simulink model "LLC_fast_PI_MOS"  (R2024a)
settings: Solver=FixedStepDiscrete  StartTime=0.0  StopTime=0.3  FixedStep=Ts_Power  RelTol=1e-3  EnableMultiTasking=on
values from neighbouring files (symbols this model uses):
  Co = 560e-6    (= 0.00056)    [LLC_Data.m]    (also in LLC_Reverse_Data.m)
  Cr = 140e-9    (= 1.4e-07)    [LLC_Data.m]    (also in LLC_Reverse_Data.m)
  fs_LCC_max = 250e3    (= 250000)    [LLC_Data.m]    (also in LLC_Reverse_Data.m)
  fs_LCC_min = 40e3    (= 40000)    [LLC_Data.m]    (also in LLC_Reverse_Data.m)
  Ki_LLC = 500e3    (= 500000)    [LLC_Data.m]    (also in LLC_Reverse_Data.m)
  Kp_LLC = 5e3    (= 5000)    [LLC_Data.m]    (also in LLC_Reverse_Data.m)
  Lm = 100e-6    (= 0.0001)    [LLC_Data.m]    (also in LLC_Reverse_Data.m)
  Lr = 20e-6    (= 2e-05)    [LLC_Data.m]    (also in LLC_Reverse_Data.m)
  Np = 11    [LLC_Data.m]    (also in LLC_Reverse_Data.m)
  Ns = 10    [LLC_Data.m]    (also in LLC_Reverse_Data.m)
  Ro = Vo_nom^2/Po_nom    (= 19.6363636364)    [LLC_Data.m]    (also in LLC_Reverse_Data.m)
  Ts_Control = 10e-6    (= 1e-05)    [LLC_Data.m]    (also in LLC_Reverse_Data.m)
  Ts_Power = 50e-9    (= 5e-08)    [LLC_Data.m]    (also in LLC_Reverse_Data.m)
  V_o_max = 450    [LLC_Data.m]    (also in LLC_Reverse_Data.m)
  V_o_min = 275    [LLC_Data.m]    (also in LLC_Reverse_Data.m)
  Vdc_in = 400    [LLC_Data.m]    (also in LLC_Reverse_Data.m)
undefined symbols (not defined in the file or in its folder): DiscIntNeverNeededParam
libraries: spsMosfetLib x8, spsVoltageMeasurementLib x5, spsOnDelayLib x4, spsSeriesRLCBranchLib x3, spsCurrentMeasurementLib x3, spsDCVoltageSourceLib x1, slpidlib x1, spsLinearTransformerLib x1, spspowerguiLib x1
settings Model: SimulationMode=accelerator  Creator=LWYohann  LastModifiedBy=LWYohann

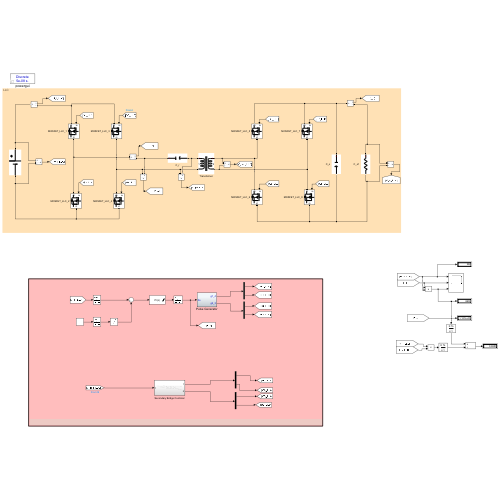
[thumbnail: Simulink's stored preview of the top-level diagram]
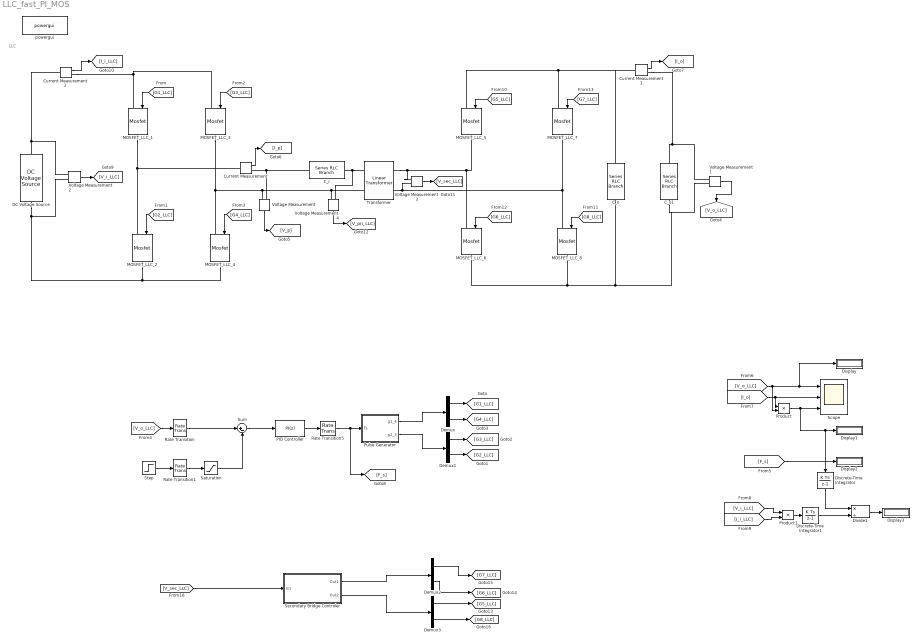
== system LLC_fast_PI_MOS ==
  note: LLC
  C_o : spsSeriesRLCBranchLib/Series RLC Branch  LConnTagsString=__new0  RConnTagsString=__new0  BranchType=C  Resistance=1  Inductance=1e-3  SetiL0=off  InitialCurrent=0  Capacitance=Co  Setx0=on  InitialVoltage=Vo_nom  Measurements=None
  C_o1 : spsSeriesRLCBranchLib/Series RLC Branch  LConnTagsString=__new0  RConnTagsString=__new0  BranchType=R  Resistance=Ro  Inductance=1e-3  SetiL0=off  InitialCurrent=0  Capacitance=Co  Setx0=on  InitialVoltage=375  Measurements=None
  C_r : spsSeriesRLCBranchLib/Series RLC Branch  LConnTagsString=__new0  RConnTagsString=__new0  BranchType=C  Resistance=1  Inductance=1e-3  SetiL0=off  InitialCurrent=0  Capacitance=Cr  Setx0=off  InitialVoltage=0  Measurements=None
  Current Measurement : spsCurrentMeasurementLib/Current Measurement  PhasorSimulation=off  OutputType=Complex  PSBequivalent=0
  Current Measurement1 : spsCurrentMeasurementLib/Current Measurement  PhasorSimulation=off  OutputType=Complex  PSBequivalent=0
  Current Measurement2 : spsCurrentMeasurementLib/Current Measurement  PhasorSimulation=off  OutputType=Complex  PSBequivalent=0
  DC Voltage Source : spsDCVoltageSourceLib/DC Voltage Source  Amplitude=Vdc_in  Measurements=None
  Demux{,1..3} (4 alike) : Demux  Outputs=2
  Discrete-Time Integrator : DiscreteIntegrator  SampleTime=Ts_Power  ICPrevOutput=DiscIntNeverNeededParam  ICPrevScaledInput=DiscIntNeverNeededParam
  Discrete-Time Integrator1 : DiscreteIntegrator  SampleTime=Ts_Power  ICPrevOutput=DiscIntNeverNeededParam  ICPrevScaledInput=DiscIntNeverNeededParam
  Display{,1..3} (4 alike) : Display
      Display3 settings: Decimation=2
  Divide1 : Product  Inputs=*/
  MOSFET_LLC_{1..8} (8 alike) : spsMosfetLib/Mosfet  Ron=Ron_FET  Lon=0  Rd=Ron_Diode  Vfd=Vf  IC=0  Rs=1e6  Cs=inf  Measurements=off
  PID Controller : slpidlib/PID Controller  Controller=PI  Form=Parallel  TimeDomain=Discrete-time  UseExternalTs=off  SampleTime=Ts_Control  IntegratorMethod=Forward Euler  FilterMethod=Forward Euler  ControllerParametersSource=internal  P=Kp_LLC  I=Ki_LLC  UseKiTs=off  D=0  UseExternalDerivativeSource=off  N=100  UseFilter=on  TunerSelectOption=Transfer Function Based (PID Tuner App)  InitialConditionSource=internal  InitialConditionForIntegrator=fr  InitialConditionForFilter=0  DifferentiatorICPrevScaledInput=0  ExternalReset=none  TrackingMode=off  Kt=1  LimitOutput=on  SatLimitsSource=internal  UpperSaturationLimit=fs_LCC_max  LowerSaturationLimit=fs_LCC_min  LinearizeAsGain=on  AntiWindupMode=none  Kb=1  LimitIntegrator=on  UpperIntegratorSaturationLimit=fs_LCC_max  LowerIntegratorSaturationLimit=fs_LCC_min  POutMin=[]  POutMax=[]  IOutMin=[]  IOutMax=[]  DOutMin=[]  DOutMax=[]  NOutMin=[]  NOutMax=[]  SumOutMin=[]  SumOutMax=[]  SaturationOutMin=[]  SaturationOutMax=[]  PParamMin=[]  PParamMax=[]  IParamMin=[]  IParamMax=[]  DParamMin=[]  DParamMax=[]  NParamMin=[]  NParamMax=[]  KbParamMin=[]  KbParamMax=[]  KtParamMin=[]  KtParamMax=[]  KbOutMin=[]  KbOutMax=[]  KtOutMin=[]  KtOutMax=[]  IntegratorOutMin=[]  IntegratorOutMax=[]  FilterOutMin=[]  FilterOutMax=[]  SumI1OutMin=[]  SumI1OutMax=[]  SumI2OutMin=[]  SumI2OutMax=[]  SumI3OutMin=[]  SumI3OutMax=[]  SumI4OutMin=[]  SumI4OutMax=[]  SumDOutMin=[]  SumDOutMax=[]  DifferentiatorOutMin=[]  DifferentiatorOutMax=[]  FilterDiffOutCoefMin=[]  FilterDiffOutCoefMax=[]  ReciprocalOutMin=[]  ReciprocalOutMax=[]  SumDenOutMin=[]  SumDenOutMax=[]  SumNumOutMin=[]  SumNumOutMax=[]  DivideOutMin=[]  DivideOutMax=[]  UdiffTsProdOutMin=[]  UdiffTsProdOutMax=[]  NTsProdOutMin=[]  NTsProdOutMax=[]  UintegralTsProdOutMin=[]  UintegralTsProdOutMax=[]  UngainTsProdOutMin=[]  UngainTsProdOutMax=[]  ClampingZeroOutDataTypeStr=Inherit: Inherit via back propagation  ClampingZeroOutMin=[]  ClampingZeroOutMax=[]  FilterDenConstantOutDataTypeStr=Inherit: Inherit via back propagation  FilterDenConstantOutMin=[]  FilterDenConstantOutMax=[]  PCopyOutDataTypeStr=Inherit: Inherit via back propagation  PCopyOutMin=[]  PCopyOutMax=[]  NCopyOutDataTypeStr=Inherit: Inherit via back propagation  NCopyOutMin=[]  NCopyOutMax=[]  IntegratorContinuousStateAttributes=''  IntegratorStateMustResolveToSignalObject=off  IntegratorRTWStateStorageClass=Auto  FilterContinuousStateAttributes=''  FilterStateMustResolveToSignalObject=off  FilterRTWStateStorageClass=Auto  ParallelPVariant=InternalParameters  IdealPVariant=Disabled  IVariant=InternalParameters  DVariant=Disabled  IntegratorVariant=Discrete  SatVariant=Enabled  AWVariant=Passthrough  PCopyVariant=Disabled  TRVariant=Disabled  FdbkBlocksVariant=Forward  IdealPFdbkVariant=Disabled  SatFdbkVariant=Disabled  DerivativeFilterVariant=Disabled  NVariant=Disabled  NCopyVariant=Disabled_SignalSpec  FilterICVariant=Disabled  IntegratorICVariant=InternalICs  ExternalResetVariant=Disabled  TRSumVariant=Passthrough  SumFdbkVariant=Disabled  SumVariant=Sum_PI  TsampFilterVariant=InternalTs  TsampNgainVariant=Passthrough  TsampIntegralVariant=Disabled_SignalSpec  ExternalSaturationOutDataTypeStr=Inherit: Same as second input  DerivativeSourceVariant=Disabled
  Product : Product
  Product1 : Product
  Pulse Generator : Subsystem
  Rate Transition : RateTransition  OutPortSampleTime=Ts_Control
  Rate Transition1 : RateTransition  OutPortSampleTime=Ts_Control
  Rate Transition5 : RateTransition  InitialCondition=fs_LCC_min  OutPortSampleTime=Ts_Power
  Saturation : Saturate  UpperLimit=V_o_max  LowerLimit=V_o_min
  Scope : Scope  NumInputPorts=3
  Secondary Bridge Controler : Subsystem
  Step : Step  Time=0.1  Before=275  After=360  SampleTime=Ts_Power
  Sum : Sum  Inputs=|+-
  Transformer : spsLinearTransformerLib/Linear Transformer  UNITS=SI  NominalPower=[ 6.6e3 100e3 ]  winding1="[Np   1e-2 Lr]"  winding2="[Ns  1e-2  1e-8 ]"  ThreeWindings=off  winding3=[3.15e+05 0.7938 0.084225]  RmLm=[1e4 Lm]  Measurements=None  DataType=on
  Voltage Measurement{,1..4} (5 alike) : spsVoltageMeasurementLib/Voltage Measurement  PhasorSimulation=off  OutputType=Complex  PSBequivalent=0
  powergui : spspowerguiLib/powergui  Priority=1  SimulationMode=Discrete  SampleTime=Ts_Power  frequency=60  Iterations=50  frequencyindice=0  Pbase=100e6  ErrMax=1e-4  UnitsV=kV  UnitsW=MW  buscounter=0  FunctionMessages=off  echomessages=off  EnableUseOfTLC=off  CurrentSourceSwitches=off  DisableSnubberDevices=off  DisableRonSwitches=off  DisableVfSwitches=off  DisplayEquations=off  AutomaticDiscreteSolvers=off  SolverType=Tustin/Backward Euler (TBE)  Interpol=off  ExternalGateDelay=off  methode=off  Ts=100  x0status=blocks  SPID=on  SwTol=0  HookPort=off  NonlinearTolerance=1e-4  nMaxIteration=100  ContinueOnMaxIteration=off  RestoreLinks=warning  ResistiveCurrentMeasurement=off  Frange=[0:2:500]  Ylog=off  Xlog=on  ShowGrid=off  save=off  variable=ZData  structure=0  ZoomFFT=off  StartTime=0.0  cycles=1  DisplayStyle=1  fundamental=60  FreqAxis=off  MaxFrequency=1000  frequencyindicesteady=1  RmsSteady=1  display=off
  wires:
  Demux/1 -> [G1_LLC]
  Demux/2 -> [G4_LLC]
  Demux1/1 -> [G3_LLC]
  Demux1/2 -> [G2_LLC]
  [G1_LLC] -> MOSFET_LLC_1/1
  [G2_LLC] -> MOSFET_LLC_2/1
  [G3_LLC] -> MOSFET_LLC_3/1
  [G4_LLC] -> MOSFET_LLC_4/1
  Voltage Measurement1/1 -> [V_o_LLC]
  [V_o_LLC] -> Rate Transition/1
  Step/1 -> Rate Transition1/1
  Rate Transition1/1 -> Saturation/1
  PID Controller/1 -> Rate Transition5/1
  Rate Transition5/1 -> [F_s], Pulse Generator/1(Fs)
  Pulse Generator/1(g1_4) -> Demux/1
  Pulse Generator/2(g2_3) -> Demux1/1
  Voltage Measurement/1 -> [V_p]
  Current Measurement/1 -> [I_p]
  Current Measurement1/1 -> [I_o]
  [V_o_LLC] -> Product/2, Display/1, Scope/1
  [I_o] -> Product/1, Scope/2
  Product/1 -> Display1/1, Discrete-Time Integrator/1, Scope/3
  [F_s] -> Display2/1
  Sum/1 -> PID Controller/1
  Rate Transition/1 -> Sum/1
  Saturation/1 -> Sum/2
  Voltage Measurement2/1 -> [V_i_LLC]
  Current Measurement2/1 -> [I_i_LLC]
  [V_i_LLC] -> Product1/1
  [I_i_LLC] -> Product1/2
  Product1/1 -> Discrete-Time Integrator1/1
  Divide1/1 -> Display3/1
  Discrete-Time Integrator/1 -> Divide1/1
  Discrete-Time Integrator1/1 -> Divide1/2
  Voltage Measurement3/1 -> [V_sec_LLC]
  [G5_LLC] -> MOSFET_LLC_5/1
  [G8_LLC] -> MOSFET_LLC_8/1
  [G6_LLC] -> MOSFET_LLC_6/1
  [G7_LLC] -> MOSFET_LLC_7/1
  Voltage Measurement4/1 -> [V_pri_LLC]
  Demux2/1 -> [G7_LLC]
  Demux3/1 -> [G5_LLC]
  Demux2/2 -> [G6_LLC]
  Demux3/2 -> [G8_LLC]
  [V_sec_LLC] -> Secondary Bridge Controler/1(In1)
  Secondary Bridge Controler/1(Out1) -> Demux2/1
  Secondary Bridge Controler/2(Out2) -> Demux3/1
  connections:
  C_r/RConn1 -- Voltage Measurement4/LConn1 -- Transformer/LConn1
  Transformer/LConn2 -- Voltage Measurement4/LConn2 -- Voltage Measurement/LConn2 -- MOSFET_LLC_4/LConn1 -- MOSFET_LLC_3/RConn1
  MOSFET_LLC_1/RConn1 -- Current Measurement/LConn1 -- MOSFET_LLC_2/LConn1
  MOSFET_LLC_3/LConn1 -- Current Measurement2/RConn1 -- MOSFET_LLC_1/LConn1
  DC Voltage Source/LConn1 -- Voltage Measurement2/LConn2 -- MOSFET_LLC_4/RConn1 -- MOSFET_LLC_2/RConn1
  Transformer/RConn1 -- Voltage Measurement3/LConn1 -- MOSFET_LLC_6/LConn1 -- MOSFET_LLC_5/RConn1
  Current Measurement1/LConn1 -- C_o/LConn1 -- MOSFET_LLC_5/LConn1 -- MOSFET_LLC_7/LConn1
  C_o/RConn1 -- C_o1/RConn1 -- Voltage Measurement1/LConn2 -- MOSFET_LLC_6/RConn1 -- MOSFET_LLC_8/RConn1
  Transformer/RConn2 -- MOSFET_LLC_8/LConn1 -- MOSFET_LLC_7/RConn1 -- Voltage Measurement3/LConn2
  C_r/LConn1 -- Voltage Measurement/LConn1 -- Current Measurement/RConn1
  Voltage Measurement1/LConn1 -- Current Measurement1/RConn1 -- C_o1/LConn1
  DC Voltage Source/RConn1 -- Current Measurement2/LConn1 -- Voltage Measurement2/LConn1

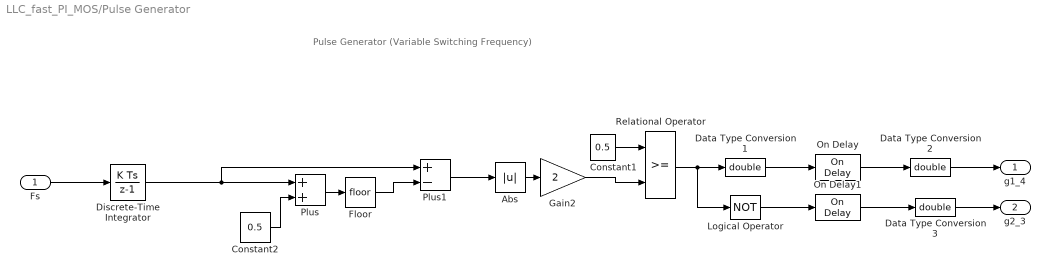
== system LLC_fast_PI_MOS/Pulse Generator ==
  note: Pulse Generator
      | (Variable Switching Frequency)
  Fs : Inport
  Abs : Abs  SaturateOnIntegerOverflow=off
  Constant1 : Constant  Value=0.5
  Constant2 : Constant  Value=0.5
  Data Type Conversion1 : DataTypeConversion  OutDataTypeStr=double  SaturateOnIntegerOverflow=off  RndMeth=Floor
  Data Type Conversion2 : DataTypeConversion  OutDataTypeStr=double  SaturateOnIntegerOverflow=off  RndMeth=Floor
  Data Type Conversion3 : DataTypeConversion  OutDataTypeStr=double  SaturateOnIntegerOverflow=off  RndMeth=Floor
  Discrete-Time Integrator : DiscreteIntegrator  SampleTime=Ts_Power  ICPrevOutput=DiscIntNeverNeededParam  ICPrevScaledInput=DiscIntNeverNeededParam
  Floor : Rounding
  Gain2 : Gain  Gain=2  SaturateOnIntegerOverflow=on  OutDataTypeStr=Inherit: Same as input  ParamDataTypeStr=Inherit: Same as input
  Logical Operator : Logic  Operator=NOT  AllPortsSameDT=off  OutDataTypeStr=float('double')
  On Delay : spsOnDelayLib/On Delay  DelayType=On delay  delay=DT_LLC  ic=0  Ts=Ts_Power
  On Delay1 : spsOnDelayLib/On Delay  DelayType=On delay  delay=DT_LLC  ic=0  Ts=Ts_Power
  Plus : Sum
  Plus1 : Sum  Inputs=+-
  Relational Operator : RelationalOperator  OutDataTypeStr=boolean  InputSameDT=off
  g1_4 : Outport  VectorParamsAs1DForOutWhenUnconnected=off
  g2_3 : Outport  Port=2  VectorParamsAs1DForOutWhenUnconnected=off
  wires:
  On Delay1/1 -> Data Type Conversion3/1
  On Delay/1 -> Data Type Conversion2/1
  Data Type Conversion1/1 -> On Delay/1
  Logical Operator/1 -> On Delay1/1
  Gain2/1 -> Relational Operator/2
  Relational Operator/1 -> Logical Operator/1, Data Type Conversion1/1
  Constant1/1 -> Relational Operator/1
  Data Type Conversion2/1 -> g1_4/1
  Data Type Conversion3/1 -> g2_3/1
  Plus/1 -> Floor/1
  Discrete-Time Integrator/1 -> Plus1/1, Plus/1
  Abs/1 -> Gain2/1
  Floor/1 -> Plus1/2
  Plus1/1 -> Abs/1
  Fs/1 -> Discrete-Time Integrator/1
  Constant2/1 -> Plus/2

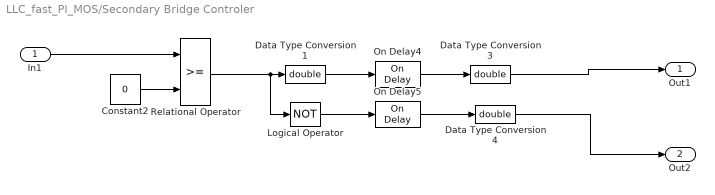
== system LLC_fast_PI_MOS/Secondary Bridge Controler ==
  In1 : Inport
  Constant2 : Constant  Value=0
  Data Type Conversion1 : DataTypeConversion  OutDataTypeStr=double  SaturateOnIntegerOverflow=off  RndMeth=Floor
  Data Type Conversion3 : DataTypeConversion  OutDataTypeStr=double  SaturateOnIntegerOverflow=off  RndMeth=Floor
  Data Type Conversion4 : DataTypeConversion  OutDataTypeStr=double  SaturateOnIntegerOverflow=off  RndMeth=Floor
  Logical Operator : Logic  Operator=NOT  AllPortsSameDT=off  OutDataTypeStr=float('double')
  On Delay4 : spsOnDelayLib/On Delay  DelayType=On delay  delay=DT_LLC  ic=0  Ts=Ts_Power
  On Delay5 : spsOnDelayLib/On Delay  DelayType=On delay  delay=DT_LLC  ic=0  Ts=Ts_Power
  Relational Operator : RelationalOperator  OutDataTypeStr=boolean  ZeroCross=off  InputSameDT=off
  Out1 : Outport
  Out2 : Outport  Port=2
  wires:
  Logical Operator/1 -> On Delay5/1
  Constant2/1 -> Relational Operator/2
  Relational Operator/1 -> Logical Operator/1, Data Type Conversion1/1
  On Delay5/1 -> Data Type Conversion4/1
  Data Type Conversion1/1 -> On Delay4/1
  On Delay4/1 -> Data Type Conversion3/1
  Data Type Conversion3/1 -> Out1/1
  Data Type Conversion4/1 -> Out2/1
  In1/1 -> Relational Operator/1
